simulink model "mpc_demo_1"  (R2019b)
settings: Solver=ode45  StartTime=0.0  StopTime=10.0  MaxStep=0.01  RelTol=1e-3  EnableMultiTasking=on
settings Model: Creator=jgillis  LastModifiedBy=Dell
settings DataIOCC: LimitDataPoints=on  SaveFormat=Array  ReturnWorkspaceOutputs=off
settings OptimizationCC: LifeSpan=inf
settings DebuggingCC: SolverPrmCheckMsg=warning  SFUnexpectedBacktrackingDiag=warning  SFNoUnconditionalDefaultTransitionDiag=warning  SFExecutionAtInitializationDiag=none  ArithmeticOperatorsInVariantConditions=warning
settings HardwareCC: ProdBitPerPointer=32  ProdBitPerSizeT=32  ProdBitPerPtrDiffT=32  ProdLargestAtomicFloat=None  ProdIntDivRoundTo=Undefined  ProdEndianess=Unspecified  ProdWordSize=32  ProdHWDeviceType=32-bit Generic
settings ModelReferenceCC: PropagateSignalLabelsOutOfModel=off
settings SFSimCC: SimUseLocalCustomCode=off  CustomCodeUndefinedFunction=UseInterfaceOnly
settings RTWCC: RTWUseLocalCustomCode=off
settings CodeAppCC: StateflowObjectComments=on
settings GRTTargetCC: TargetLangStandard=C89/C90 (ANSI)  GeneratePreprocessorConditionals=Disable all
settings ConfigComp: CovMetricSettings=dw  CovHtmlReporting=on  CovSaveCumulativeToWorkspaceVar=on  CovSaveSingleToWorkspaceVar=on  CovExternalEMLEnable=off  CovSFcnEnable=off

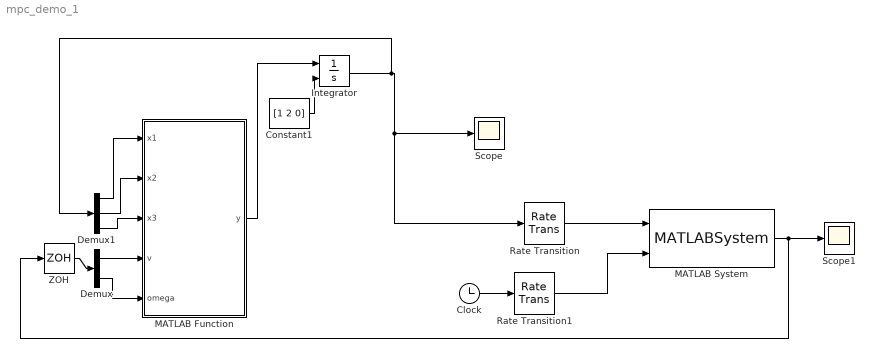
== system mpc_demo_1 ==
  Clock : Clock
  Constant1 : Constant  Value=[1 2 0]
  Demux : Demux  Outputs=2
  Demux1 : Demux  Outputs=3
  Integrator : Integrator  InitialConditionSource=external  InitialCondition=[1 0]'
  MATLAB Function : MATLAB Function  TreatAsAtomicUnit=on
  MATLAB System : MATLABSystem  System=single_robot_controller  SimulateUsing=Interpreted execution
      mask Type: single_robot_controller
      mask Display:
      | disp('single_robot_controller');
      | port_label('input',1,'x');
      | port_label('input',2,'t');
      | port_label('output',1,'u');
  Rate Transition : RateTransition  OutPortSampleTime=0.5
  Rate Transition1 : RateTransition  OutPortSampleTime=0.5
  Scope : Scope
  Scope1 : Scope
  ZOH : ZeroOrderHold  SampleTime=0.5
  wires:
  Integrator/1 -> Demux1/1, Rate Transition/1, Scope/1
  Constant1/1 -> Integrator/2
  MATLAB System/1 -> Scope1/1, ZOH/1
  Clock/1 -> Rate Transition1/1
  Rate Transition/1 -> MATLAB System/1
  Rate Transition1/1 -> MATLAB System/2
  MATLAB Function/1(y) -> Integrator/1
  ZOH/1 -> Demux/1
  Demux/1 -> MATLAB Function/4(v)
  Demux/2 -> MATLAB Function/5(omega)
  Demux1/1 -> MATLAB Function/1(x1)
  Demux1/2 -> MATLAB Function/2(x2)
  Demux1/3 -> MATLAB Function/3(x3)

== matlab function mpc_demo_1/MATLAB Function ==
  data: y output; x1 input; x2 input; x3 input; v input; omega input
function y = rhs(x1,x2,x3,v,omega)
%#codegen

y = [v*cos(x3);v*sin(x3);omega];


end
